simulink subsystem "Pilot_arm"  (R2024a)
settings: Solver=VariableStepAuto  StartTime=0.0  StopTime=10.0  RelTol=1e-3
libraries: simulink x1
settings Model: Creator=gurt1  LastModifiedBy=gurt1

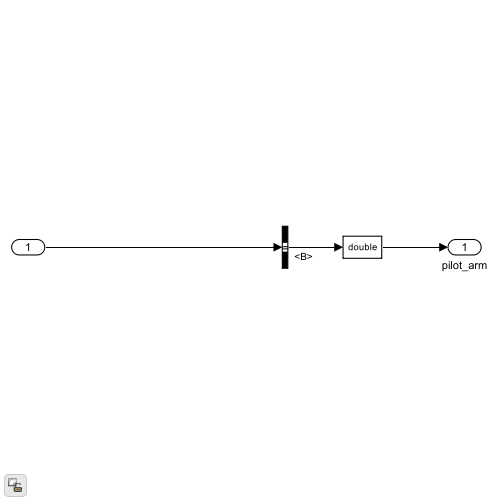
[thumbnail: Simulink's stored preview of the top-level diagram]
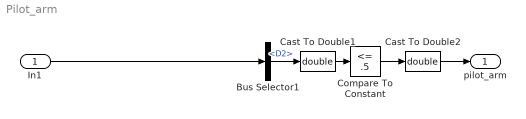
== system Pilot_arm ==
  In1 : Inport
  Bus Selector1 : BusSelector  OutputSignals=switches.D2
  Cast To Double1 : DataTypeConversion  OutDataTypeStr=double  SaturateOnIntegerOverflow=off  RndMeth=Floor
  Cast To Double2 : DataTypeConversion  OutDataTypeStr=double  SaturateOnIntegerOverflow=off  RndMeth=Floor
  Compare To Constant : simulink/Logic and Bit Operations/Compare To Constant  relop=<=  const=.5  OutDataTypeStr=boolean
  pilot_arm : Outport
  wires:
  Bus Selector1/1 -> Cast To Double1/1  "<D2>"
  In1/1 -> Bus Selector1/1
  Cast To Double1/1 -> Compare To Constant/1
  Compare To Constant/1 -> Cast To Double2/1
  Cast To Double2/1 -> pilot_arm/1
